simulink model "plant_VV"  (R2023a)
settings: Solver=FixedStepAuto  StartTime=0.0  StopTime=10.0  FixedStep=0.01  RelTol=1e-3
undefined symbols (not defined in the file or in its folder): g, m, sys
libraries: simulink_extras x4, shared6dof x1
settings Model: Creator=timme  LastModifiedBy=timme
settings OptimizationCC: BlockReduction=off  DefaultParameterBehavior=Inlined  BufferReuse=off

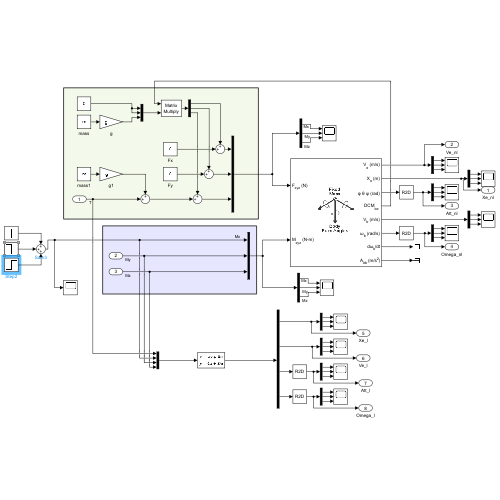
[thumbnail: Simulink's stored preview of the top-level diagram]
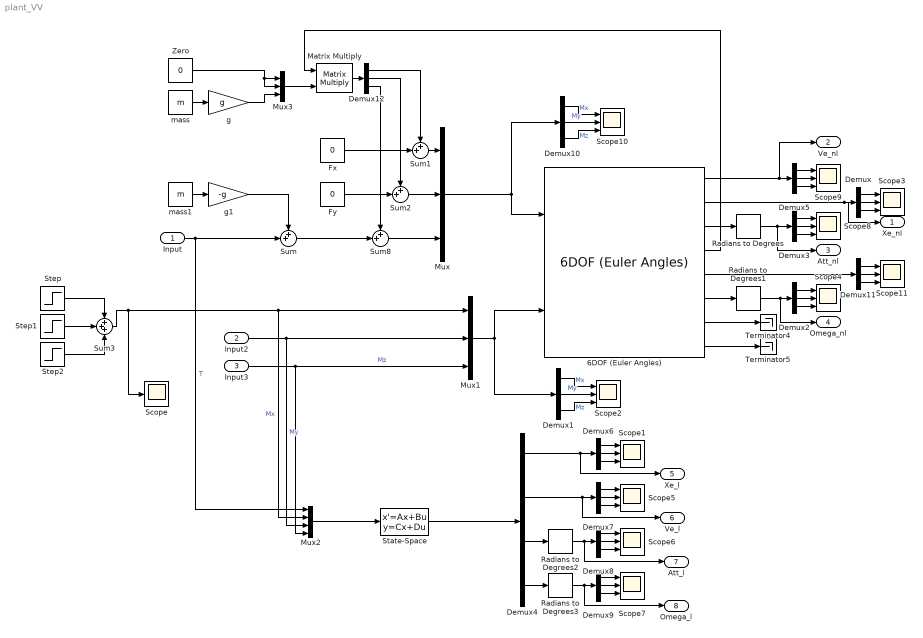
== system plant_VV ==
  Input : Inport
  Input2 : Inport  Port=2
  Input3 : Inport  Port=3
  6DOF (Euler Angles) : shared6dof/6DOF (Euler Angles)  units=Metric (MKS)  mtype=Fixed  rep=Euler Angles  xme_0=[0 0 0]  Vm_0=[0 0 0]  eul_0=[0 0 0]  pm_0=[0 0 0]  mass_0=m  mass_e=0.5  mass_f=2.0  inertia=I  inertia_e=eye(3)  inertia_f=2*eye(3)  k_quat=1.0  vre_flag=on  abi_flag=off  aMode=0  xme_statename=''  Vm_statename=''  eul_statename=''  quat_statename=''  pm_statename=''  mass_statename=''
  Demux{,1..3,5..12} (12 alike) : Demux  Outputs=3
  Demux4 : Demux  Outputs=[3 3 3 3]
  Fx : Constant  Value=0
  Fy : Constant  Value=0
  Matrix Multiply : Product  Inputs=**  Multiplication=Matrix(*)
  Mux : Mux  Inputs=3
  Mux1 : Mux  Inputs=3
  Mux2 : Mux
  Mux3 : Mux  Inputs=3
  Radians to Degrees{,1..3} (4 alike) : simulink_extras/Transformations/Radians to Degrees
  Scope : Scope
  Scope{1..11} (11 alike) : Scope  NumInputPorts=3
  State-Space : StateSpace  A=sys.A  B=sys.B  C=sys.C  D=sys.D  InitialCondition=0
  Step : Step  Time=0.05  Before=0.2  After=0  SampleTime=0
  Step1 : Step  Time=0.05  After=-0.2  SampleTime=0
  Step2 : Step  Time=0.1  After=0.2  SampleTime=0
  Sum{,1..2,8} (4 alike) : Sum  Inputs=++|
  Sum3 : Sum  Inputs=+++
  Terminator4 : Terminator
  Terminator5 : Terminator
  Zero : Constant  Value=0  OutDataTypeStr=Inherit: Inherit via back propagation
  g : Gain  Gain=g
  g1 : Gain  Gain=-g
  mass : Constant  Value=m
  mass1 : Constant  Value=m
  Xe_nl : Outport
  Ve_nl : Outport  Port=2
  Att_nl : Outport  Port=3
  Omega_nl : Outport  Port=4
  Xe_l : Outport  Port=5
  Ve_l : Outport  Port=6
  Att_l : Outport  Port=7
  Omega_l : Outport  Port=8
  wires:
  Fx/1 -> Sum1/2
  Fy/1 -> Sum2/2
  Mux1/1 -> 6DOF (Euler Angles)/2, Demux1/1
  Demux1/2 -> Scope2/2  "My"
  Demux1/1 -> Scope2/1  "Mx"
  Demux1/3 -> Scope2/3  "Mz"
  Sum8/1 -> Mux/3
  Sum3/1 -> Mux2/2, Mux1/1, Scope/1  "Mx"
  Input3/1 -> Mux2/4, Mux1/3  "Mz"
  Input/1 -> Sum/2, Mux2/1  "T"
  Demux7/2 -> Scope5/2
  Demux4/2 -> Ve_l/1, Demux7/1
  Demux7/3 -> Scope5/3
  Demux6/2 -> Scope1/2
  Radians to Degrees3/1 -> Omega_l/1, Demux9/1
  Demux9/1 -> Scope7/1
  State-Space/1 -> Demux4/1
  Demux9/2 -> Scope7/2
  Demux8/1 -> Scope6/1
  Demux4/3 -> Radians to Degrees2/1
  Demux4/4 -> Radians to Degrees3/1
  Demux6/3 -> Scope1/3
  Demux7/1 -> Scope5/1
  Radians to Degrees2/1 -> Att_l/1, Demux8/1
  Demux6/1 -> Scope1/1
  Demux9/3 -> Scope7/3
  Demux4/1 -> Xe_l/1, Demux6/1
  Demux8/3 -> Scope6/3
  Demux8/2 -> Scope6/2
  6DOF (Euler Angles)/8 -> Terminator5/1
  Demux2/1 -> Scope4/1
  Demux5/1 -> Scope9/1
  6DOF (Euler Angles)/5 -> Demux11/1
  6DOF (Euler Angles)/2 -> Xe_nl/1, Demux/1
  Radians to Degrees1/1 -> Omega_nl/1, Demux2/1
  Demux5/2 -> Scope9/2
  6DOF (Euler Angles)/6 -> Radians to Degrees1/1
  Demux3/2 -> Scope8/2
  6DOF (Euler Angles)/4 -> Matrix Multiply/1
  Demux/3 -> Scope3/3
  Demux/2 -> Scope3/2
  Demux3/3 -> Scope8/3
  Demux/1 -> Scope3/1
  Demux2/3 -> Scope4/3
  Demux3/1 -> Scope8/1
  6DOF (Euler Angles)/7 -> Terminator4/1
  Demux5/3 -> Scope9/3
  6DOF (Euler Angles)/3 -> Radians to Degrees/1
  Radians to Degrees/1 -> Att_nl/1, Demux3/1
  Demux2/2 -> Scope4/2
  Mux2/1 -> State-Space/1
  Demux10/2 -> Scope10/2  "My"
  Demux10/1 -> Scope10/1  "Mx"
  Mux/1 -> Demux10/1, 6DOF (Euler Angles)/1
  Demux10/3 -> Scope10/3  "Mz"
  Demux11/2 -> Scope11/2
  Demux11/3 -> Scope11/3
  Demux11/1 -> Scope11/1
  g/1 -> Mux3/3
  mass/1 -> g/1
  Matrix Multiply/1 -> Demux12/1
  Sum1/1 -> Mux/1
  Demux12/1 -> Sum1/1
  Sum2/1 -> Mux/2
  Demux12/2 -> Sum2/1
  Demux12/3 -> Sum8/1
  Zero/1 -> Mux3/1, Mux3/2
  Mux3/1 -> Matrix Multiply/2
  Input2/1 -> Mux2/3, Mux1/2  "My"
  6DOF (Euler Angles)/1 -> Ve_nl/1, Demux5/1
  g1/1 -> Sum/1
  Sum/1 -> Sum8/2
  mass1/1 -> g1/1
  Step/1 -> Sum3/1
  Step1/1 -> Sum3/2
  Step2/1 -> Sum3/3
